simulink model "linnonlin"  (R2015a)
settings: Solver=ode45  StartTime=0.0  StopTime=100.0  RelTol=1e-3
values from neighbouring files (symbols this model uses):
  A = [-14.6713035715  4.37250120377; 876.704382024  -262.351072226]    [Correcteur.mat]    (also in DVinitialisation.m = [[(mufre*cxe-ba-brr)/m nfre*cxe/m];     [-r0*mufre*cxe/Jr -r; Fct_transfer_lineaire.m = [[a1 a2];     a3 a4]; QFT.m = [[(mufre*cxe-ba-brr)/m nu*cxe/m];[-r0*mufre*cxe/J -r0*nu*cxe)
  B = [0 -125]    [Correcteur.mat]    (also in DVinitialisation.m = [0;-K/Jr]; Fct_transfer_lineaire.m = [0;K]; QFT.m = [0;-K/J]; pacejka_BE_Matlab_fnc.m = BCD/(C*D))
  C = [0 1]    [Correcteur.mat]    (also in DVinitialisation.m; Fct_transfer_lineaire.m; QFT.m; pacejka_BE_Matlab_fnc.m = C_0)
  D = 0    [Correcteur.mat]    (also in DVinitialisation.m = [0]; Fct_transfer_lineaire.m = [0]; QFT.m = [0]; QFTsynth.m = max(step(K*Gn/(1+K*G))))
  W0 = 64.9781778438    [Correcteur.mat]    (also in DVinitialisation.m = 1/r0*(Vx0/(1-(Te/100))); QFT.m = 1/r0*(Vx0/(1-(Te/100))))
libraries: cstblocks x1
settings Model: Creator=StephaneBarroso  LastModifiedBy=StephaneBarroso

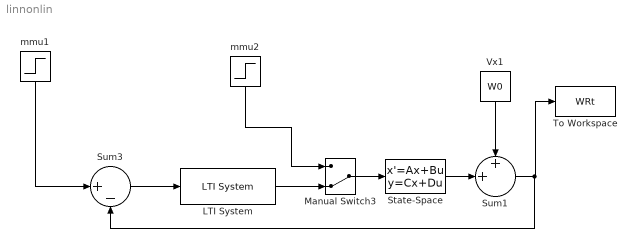
== system linnonlin ==
  LTI System : cstblocks/LTI System  sys=Correcteur  IC=[]
  Manual Switch3 : ManualSwitch  CurrentSetting=0
  State-Space : StateSpace  A=A  B=B  C=C  D=D  X0=0
  Sum1 : Sum  Inputs=++|
  Sum3 : Sum  Inputs=|+-
  To Workspace : ToWorkspace  VariableName=WRt  SaveFormat=Timeseries  SampleTime=-1
  Vx1 : Constant  Value=W0
  mmu1 : Step  Time=5  Before=W0  After=W0-5  SampleTime=0
  mmu2 : Step  Time=5  After=0.043  SampleTime=0
  wires:
  Sum3/1 -> LTI System/1
  LTI System/1 -> Manual Switch3/2
  mmu2/1 -> Manual Switch3/1
  mmu1/1 -> Sum3/1
  Manual Switch3/1 -> State-Space/1
  State-Space/1 -> Sum1/2
  Vx1/1 -> Sum1/1
  Sum1/1 -> Sum3/2, To Workspace/1
